simulink subsystem "Gcm_non_lin"  (R2021b)
settings: Solver=VariableStepAuto  StartTime=0.0  StopTime=10.0  RelTol=1e-3
values from neighbouring files (symbols this model uses):
  Gcm = numden2system(Gcm_num, Gcm_den)    [Main.m]    (also in Main_plaque_sphere.m; Main_poutre_sphere.m)
  K_SM_3 = nm*kt*Kg*ng    (= 0.33398001)    [Main.m]    (also in Main_plaque_sphere.m; Main_poutre_sphere.m)
settings Model: Creator=sama1402  LastModifiedBy=levm1106

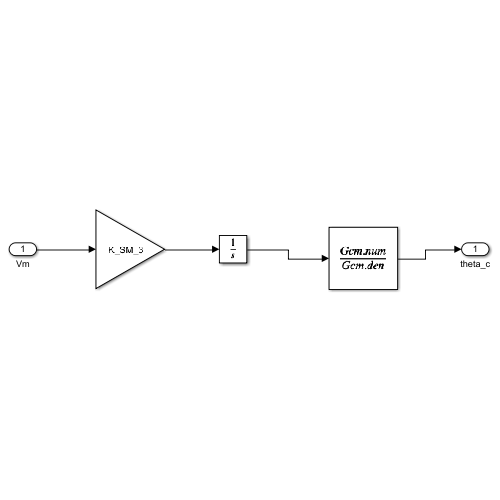
[thumbnail: Simulink's stored preview of the top-level diagram]
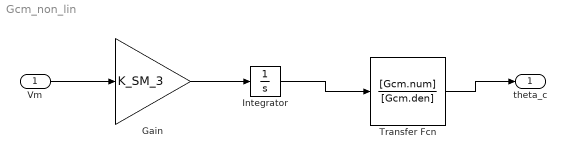
== system Gcm_non_lin ==
  Vm : Inport
  Gain : Gain  Gain=K_SM_3
  Integrator : Integrator
  Transfer Fcn : TransferFcn  Numerator=[Gcm.num]  Denominator=[Gcm.den]
  theta_c : Outport
  wires:
  Transfer Fcn/1 -> theta_c/1
  Integrator/1 -> Transfer Fcn/1
  Gain/1 -> Integrator/1
  Vm/1 -> Gain/1
